simulink model "vodarna_model"  (R2012b)
settings: Solver=ode45  StartTime=0.0  StopTime=350  MaxStep=1e-2  MinStep=1e-3  RelTol=1e-3
values from neighbouring files (symbols this model uses):
  C1 = 6.1228e-6    (= 6.1228e-06)    [iniFINAL.m]
  C2 = C1    (= 6.1228e-06)    [iniFINAL.m]
  C3 = 4.0856e-5    (= 4.0856e-05)    [iniFINAL.m]
  G = 9500    [iniFINAL.m]
  G2 = 0.04    [iniFINAL.m]
  I = 15.6e-3    (= 0.0156)    [iniFINAL.m]
  R1 = 0.1    [iniFINAL.m]
  R2 = 1.3871e+7    (= 13871000)    [iniFINAL.m]
  R3 = 5.2401e+6    (= 5240100)    [iniFINAL.m]
  R4 = 1.0172e7    (= 10172000)    [iniFINAL.m]
  R5 = R1    (= 0.1)    [iniFINAL.m]
  T = 21.5    [iniFINAL.m]
settings Model: Creator=SerzaNT  LastModifiedBy=SerzaNT

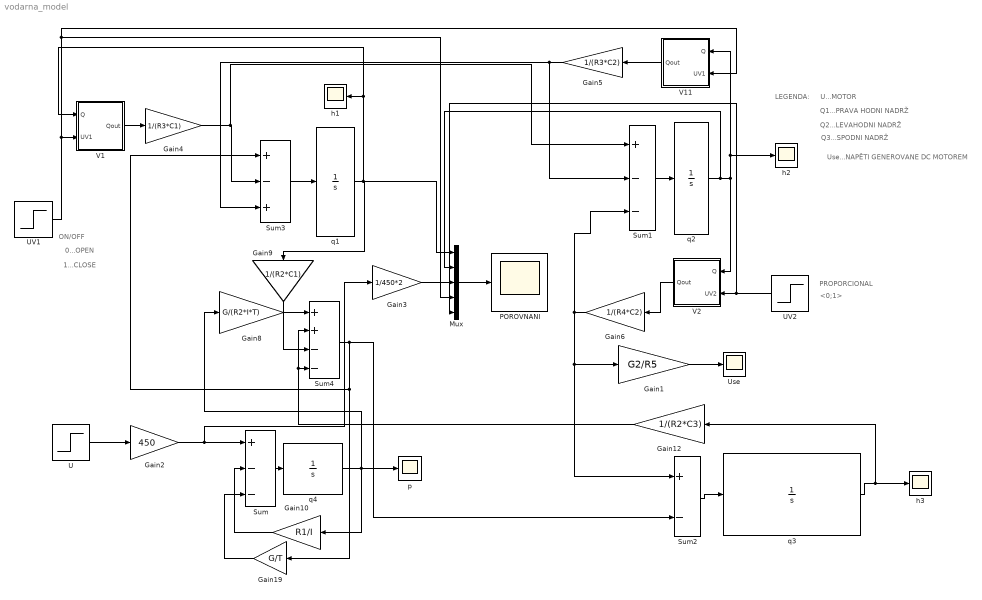
== system vodarna_model ==
  note: <0;1>
  note: PROPORCIONAL
  note: 1...CLOSE
  note: 0...OPEN
  note: ON/OFF
  note: Use...NAPĚTI GENEROVANE DC MOTOREM
  note: LEGENDA:
  note: U...MOTOR
  note: Q1...PRAVA HODNI NADRŽ
  note: Q2...LEVAHODNI NADRŽ
  note: Q3...SPODNI NADRŽ
  Gain1 : Gain  Gain=G2/R5
  Gain10 : Gain  Gain=R1/I
  Gain12 : Gain  Gain=1/(R2*C3)
  Gain19 : Gain  Gain=G/T
  Gain2 : Gain  Gain=450
  Gain3 : Gain  Gain=1/450*2
  Gain4 : Gain  Gain=1/(R3*C1)
  Gain5 : Gain  Gain=1/(R3*C2)
  Gain6 : Gain  Gain=1/(R4*C2)
  Gain8 : Gain  Gain=G/(R2*I*T)
  Gain9 : Gain  Gain=1/(R2*C1)
  Mux : Mux  Inputs=5
  "POROVNANI " : Scope
      settings: TimeRange=350  YMin=0  YMax=0.014
  Sum : Sum  Inputs=+--
  Sum1 : Sum  Inputs=+--
  Sum2 : Sum  Inputs=+-
  Sum3 : Sum  Inputs=+-+
  Sum4 : Sum  Inputs=++--
  U : Step  Time=120  Before=1  After=0  SampleTime=0
  UV1 : Step  Time=50  Before=1  After=0  SampleTime=0
  UV2 : Step  Time=250  SampleTime=0
  Use : Scope
      settings: SaveName=h
  V1 : Subsystem
      mask Display: image(imread('V1.png'))
  V11 : Subsystem
      mask Display: image(imread('V1.png'))
  V2 : Subsystem
      mask Display: image(imread('V2.png'))
  h1 : Scope
  h2 : Scope
      settings: SaveName=ScopeData2
  h3 : Scope
      settings: SaveName=h1
  p : Scope
      settings: SaveName=ScopeData4
  q1 : Integrator  LimitOutput=on  LowerSaturationLimit=0
      mask Display: image(imread('Q1.png'))
  q2 : Integrator  LimitOutput=on  LowerSaturationLimit=0
      mask Display: image(imread('Q2.png'))
  q3 : Integrator  InitialCondition=10  LimitOutput=on  LowerSaturationLimit=0
      mask Display: image(imread('Q3.png'))
  q4 : Integrator
      mask Display: image(imread('P.png'))
  wires:
  Sum1/1 -> q2/1
  Sum2/1 -> q3/1
  q3/1 -> Gain12/1, h3/1
  Mux/1 -> "POROVNANI "/1
  Sum/1 -> q4/1
  Sum3/1 -> q1/1
  Sum4/1 -> Sum2/2, Sum3/1, Gain19/1
  Gain4/1 -> Sum1/1, Sum3/2
  Gain1/1 -> Use/1
  UV1/1 -> Mux/4, V11/2(UV1), V1/2(UV1)
  UV2/1 -> Mux/5, V2/2(UV2)
  q4/1 -> p/1, Gain8/1, Gain10/1
  Gain10/1 -> Sum/2
  U/1 -> Gain2/1
  Gain8/1 -> Sum4/1
  Gain12/1 -> Sum4/4, Sum4/2
  q1/1 -> V1/1(Q), h1/1, Mux/1, Gain9/1
  Gain9/1 -> Sum4/3
  Gain19/1 -> Sum/3
  q2/1 -> Mux/2, h2/1, V11/1(Q), V2/1(Q)
  V2/1(Qout) -> Gain6/1
  V1/1(Qout) -> Gain4/1
  V11/1(Qout) -> Gain5/1
  Gain5/1 -> Sum1/2, Sum3/3
  Gain6/1 -> Gain1/1, Sum2/1, Sum1/3
  Gain2/1 -> Gain3/1, Sum/1
  Gain3/1 -> Mux/3

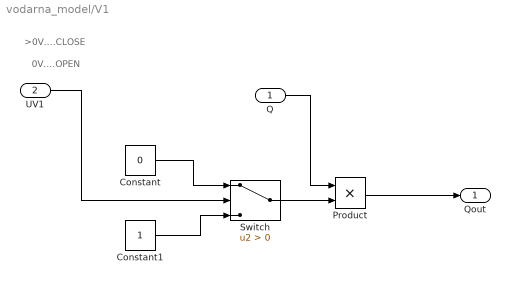
== system vodarna_model/V1 ==
  note: >0V....CLOSE
  note: 0V....OPEN
  Q : Inport
  UV1 : Inport  Port=2
  Constant : Constant  Value=0
  Constant1 : Constant
  Product : Product  RndMeth=Zero
  Switch : Switch  Criteria=u2 > Threshold
  Qout : Outport
  wires:
  Q/1 -> Product/1
  Product/1 -> Qout/1
  UV1/1 -> Switch/2
  Constant/1 -> Switch/1
  Constant1/1 -> Switch/3
  Switch/1 -> Product/2

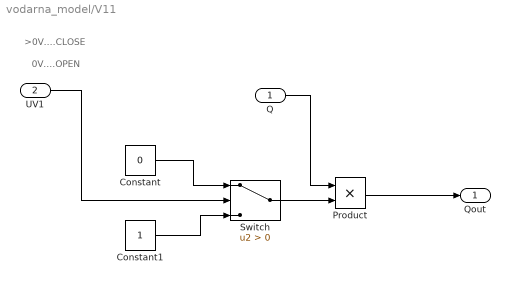
== system vodarna_model/V11 ==
  note: 0V....OPEN
  note: >0V....CLOSE
  Q : Inport
  UV1 : Inport  Port=2
  Constant : Constant  Value=0
  Constant1 : Constant
  Product : Product  RndMeth=Zero
  Switch : Switch  Criteria=u2 > Threshold
  Qout : Outport
  wires:
  Switch/1 -> Product/2
  Constant1/1 -> Switch/3
  Constant/1 -> Switch/1
  UV1/1 -> Switch/2
  Product/1 -> Qout/1
  Q/1 -> Product/1

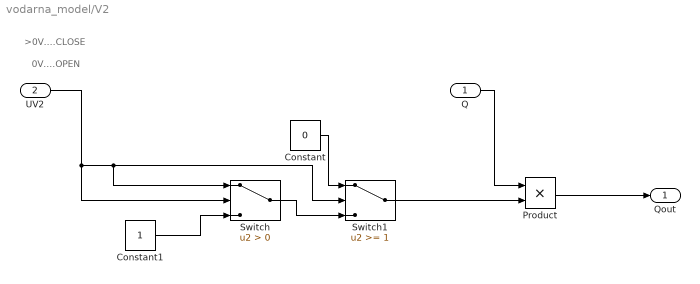
== system vodarna_model/V2 ==
  note: >0V....CLOSE
  note: 0V....OPEN
  Q : Inport
  UV2 : Inport  Port=2
  Constant : Constant  Value=0
  Constant1 : Constant
  Product : Product  RndMeth=Zero
  Switch : Switch  Criteria=u2 > Threshold
  Switch1 : Switch  Threshold=1
  Qout : Outport
  wires:
  Q/1 -> Product/1
  Product/1 -> Qout/1
  UV2/1 -> Switch/2, Switch/1, Switch1/2
  Constant1/1 -> Switch/3
  Constant/1 -> Switch1/1
  Switch/1 -> Switch1/3
  Switch1/1 -> Product/2
